simulink model "OpenLoopSpacecraft"  (Simulink 7.4)
settings: Solver=ode5  StartTime=0  StopTime=30  FixedStep=DeltaT  RelTol=1e-3
InitFcn:
  | %Bifocal Relay Mirror Spacecraft Dynamics Simulation          TA Sands
  | clear all;close all;clc;
  | 
  | %Constants0
  | Re=6371.2e3;mu=398601.2e9;          %earth radius and universal gravitation constant
  | 
  | %Spacecraft orbit
  | h=0;                                     %orbit altitude
  | R=Re+h;                             %orbit radius from center of earth
  | we=0.000072921158553;   %earth's angular velocity rad/solar sec(Vallado)
  | wo=sqrt(mu/(Re+h)^3);        %orbit angular velocity
  | incln=36.6001*pi/180;          %Inclination assumed Monterey Latitude
  | epsilon=12*pi/180;  alphao=0;
  | uo=0; nuo=0;                        %Start S/C beneath subsolar point
  | beta=60; gamma=1.5;
  | a=0.545491852; b=0.314939867;  c=0.704226952;   %Assumed spacecraft rectangular size
  | Area=[b*c a*c a*b];                 %projected area~m^2 in body x,y,z directions
  | density=4.39e-14;
  | kpre=-9.9639/24/3600/180*pi*0;      %nodal precession constant assumed zero here
  | wn=kpre*(Re/(Re+h))^3.5*cos(incln); %nodal precession (zero eccentricity)
  | V=wo*(Re+h);
  | rho=asin(Re/(h+Re));                %earth angular radius
  | Cd=2.5;     psun=4.5E-6;            %Drag coefficient and solar pressure constant~N/m^2
  | Kaero=-0.5*Cd*V^2;   Psolar=2*psun;  %constants for aero and solar torque calculation
  | dL=[0.002 0.002 0.008];             %predicted distance between cp and cg
  | Kme=2.3390e-005;
  | 
  | %Spacecraft Magnetic Properties (assumed)
  | mresid=[0 0 0.01];                  %Spacecraft residual magnetic moment
  | M=mresid;                           %Magnetic unit dipole vector
  | K=7.943e15;
  | 
  | %Spacecraft Inertia conditions
  | Ix=119.1259;   Iy=150.6615;   Iz=106.0288;  Ixy=-15.7678;  Iyz=22.31637;  Ixz=-6.54859;
  | Jact=[Ix Ixy Ixz;        Ixy  Iy  Iyz;       Ixz Iyz  Iz];                  %Moment of inertia matrix
  | 
  | Ix=90;   Iy=100;   Iz=250 ;   Ixy=10;  Iyz=-20;  Ixz=10;
  | Imo=[Ix Ixy Ixz;        Ixy  Iy  Iyz;       Ixz Iyz  Iz]                  %Moment of inertia matrix
  | %Jact=Imo
  | Iinv=(Imo)^-1                      %Moment of inertia inverse goes in dynamics block
  | 
  | %Spacecraft initial Euler state angles and rates
  | phio=0;thetao=0;psio=0;                    %Initial Euler Angles
  | phidoto=0;thetadoto=0;psidoto=0;     %Initial Euler Rates
  | 
  | %Calculation of initial quaternion (qo) and angular momentum (Ho)
  | s1=sin(phio/2);s2=sin(thetao/2);s3=sin(psio/2);c1=cos(phio/2);c2=cos(thetao/2);c3=cos(psio/2);
  | q1o=s1*c2*c3-c1*s2*s3;
  | q2o=c1*s2*c3+s1*c2*s3;              %Wie pg. 321
  | q3o=c1*c2*s3-s1*s2*c3;
  | q4o=c1*c2*c3+s1*s2*s3;
  | S1=sin(phio);S2=sin(thetao);S3=sin(psio);C1=cos(phio);C2=cos(thetao);C3=cos(psio);
  | wxo=phidoto-psidoto*S2-wo*S3*C2;
  | wyo=thetadoto*C1+psidoto*C2*S1-wo*(C3*C1+S3*S2*S1);
  | wzo=psidoto*C2*C1-thetadoto*S1-wo*(S3*S2*C1-C3*S1);
  | qo=[q1o q2o q3o q4o];
  | Ho=Imo*[wxo wyo wzo]';
  | norm(Ho)*1000;
  | 
  | %Calculate eclipse time for comparison with EPS calculations
  | Te=100.87*2*V/2/pi;
  | 
  | %CMG Properties (in degrees)
  | %beta=90*pi/180;                                     %Skew angle in degrees converted to radians
  | beta=[90;90;-90;0]; beta=beta.*pi./180;
  | 
  | Gimbal0=[-30*pi/180; 90*pi/180; -30*pi/180;0];   % Initial Gimbal angles for 0 H spin up
  | w_wheel=2800*(2*pi/60);                       %Wheel speed in RPM converted to rad/s
  | Iwheel=0.0614*1.3558179483314;        % Wheel inertia in slug-ft^2 converted (exact) to kg m^2
  | h_wheel=Iwheel*w_wheel;                     % CMG Wheel Angular Momentum
  | 
  | %PID Controller Gains
  | Kpx=100;   Kdx=300;   Kix=0;  Kpy=Kpx;   Kdy=Kdx;   Kiy=Kix;  Kpz=Kpx;   Kdz=Kdx;   Kiz=Kix;
  | %Kpx=10100;   Kdx=1.6*Kpx;   Kix=0;  Kpy=Kpx;   Kdy=Kdx;   Kiy=Kix;  Kpz=Kpx;   Kdz=Kdx;   Kiz=Kix;
  | Kff=-1;
  | roll=0;  pitch=0; yaw=30;   roll=roll*pi/180; pitch=pitch*pi/180; yaw=yaw*pi/180;
  | SlewTime=10;  Rate=40;   DeltaT=1/Rate;   SPUDengage=0 ; %yaw*180/pi/100000
  | 
  | % Adaptive feedforward parameters
  | ETA=7;  ETAc=1;
  | Ix=119.1259;   Iy=150.6615;   Iz=106.0288;  Ixy=-15.7678;  Iyz=22.31637;  Ixz=-6.54859; Imo;
  | Jhat0=[Ix Ixy Ixz;       Ixy  Iy  Iyz;       Ixz Iyz  Iz];
  | ThetaHat0=[Ix; Ixy; Ixz; Iy; Iyz; Iz; 0; 0; 0];
StopFcn:
  | figure(1);subplot(3,1,1);plot(t,JwdotCMD,'linewidth',2);grid;ylabel('FeedForward','fontname','time','fontsize',20)
  | title('FeedForward Trajectory No Disturbance','fontname','time','fontsize',20);legend('roll \phi','pitch \theta','yaw \psi')
  | subplot(3,1,2);plot(t,Jwdot,'linewidth',2);grid;ylabel('Output','fontname','time','fontsize',20)
  | subplot(3,1,3);plot(t,Jwdot-JwdotCMD,'linewidth',2);grid;ylabel('Trajectory Error','fontname','time','fontsize',20)
  | xlabel('time(sec)','fontname','time','fontsize',20);
libraries: aerospace x2, simulink x1
settings Model: Creator=tasands  LastModifiedBy=tasands
settings DataIOCC: SignalLoggingName=sigsOut
settings OptimizationCC: InlineInvariantSignals=on  InitFltsAndDblsToZero=on
settings DebuggingCC: SaveWithParameterizedLinksMsg=none  SignalResolutionControl=TryResolveAllWithWarning  SolverPrmCheckMsg=none  MultiTaskDSMMsg=warning  MultiTaskCondExecSysMsg=none  StrictBusMsg=None
settings HardwareCC: TargetHWDeviceType=32-bit Generic  ProdEqTarget=off
settings RTWCC: IncludeERTFirstTime=on
settings GRTTargetCC: TargetFcnLib=ansi_tfl_tmw.mat

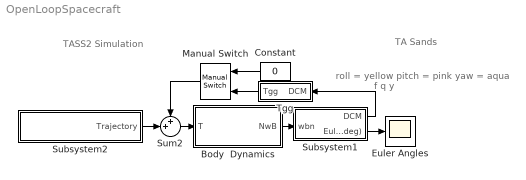
== system OpenLoopSpacecraft ==
  note: roll = yellow
      | pitch = pink
      | yaw = aqua
  note: TASS2 Simulation
  note: TA Sands
  note: f
      | q
      | y
  Body  Dynamics : Subsystem
      mask Display: disp('TASS2 Dynamics')
  Constant : Constant  Value=0  OutDataType=sfix(16)  OutScaling=2^0
  Euler Angles : Scope
      settings: TimeRange=30  YMin=-20  YMax=100
  Manual Switch : simulink/Signal Routing/Manual Switch  SystemSampleTime=-1  sw=1  action=0  varsize=off
  Subsystem1 : Subsystem
      mask Display: disp('Kinematics')
  Subsystem2 : Subsystem
      mask Display: disp('FeedForward Trajectory')
  Sum2 : Sum  Inputs=++|  OutDataType=sfix(16)  OutScaling=2^0  SaturateOnIntegerOverflow=on
  Tgg : Subsystem
      mask Display: disp('CG offet')
  wires:
  Body  Dynamics/1(NwB) -> Subsystem1/1(wbn)
  Subsystem1/1(DCM) -> Tgg/1(DCM)
  Subsystem1/2(Euler(deg)) -> Euler Angles/1
  Sum2/1 -> Body  Dynamics/1(T)
  Subsystem2/1(Trajectory) -> Sum2/2
  Manual Switch/1 -> Sum2/1
  Tgg/1(Tgg) -> Manual Switch/2
  Constant/1 -> Manual Switch/1

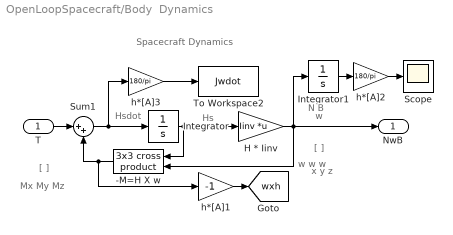
== system OpenLoopSpacecraft/Body  Dynamics ==
  note: w
  note: N B
  note: Hs
  note: Hsdot
  note: [ ]
  note: Mx
      | My
      | Mz
  note: [ ]
  note: w
      | w
      | w
  note: x
      | y
      | z
  note: Spacecraft Dynamics
  T : Inport  OutDataType=sfix(16)  OutScaling=2^0
  -M=H X w : aerospace/Axes Transformations/3x3 cross product  SystemSampleTime=-1
  H * Iinv : Gain  Gain=Iinv  Multiplication=Matrix(K*u)  ParameterDataType=sfix(16)  ParameterScaling=2^0  OutDataType=sfix(16)  OutScaling=2^0  SaturateOnIntegerOverflow=on  OutDataTypeStr=Inherit: Same as input  ParamDataTypeStr=Inherit: Same as input
  Integrator : Integrator
  Integrator1 : Integrator
  Scope : Scope
      settings: TimeRange=30  YMin=-50  YMax=200  SaveName=ScopeData5
  Sum1 : Sum  Inputs=|++  OutDataType=sfix(16)  OutScaling=2^0  SaturateOnIntegerOverflow=on  InputSameDT=on  OutDataTypeStr=Inherit: Same as first input
  To Workspace2 : ToWorkspace  VariableName=Jwdot  SampleTime=-1  SaveFormat=Array
  h*[A]1 : Gain  Gain=-1  ParameterDataType=sfix(16)  ParameterScaling=2^0  OutDataType=sfix(16)  OutScaling=2^0
  h*[A]2 : Gain  Gain=180/pi  ParameterDataType=sfix(16)  ParameterScaling=2^0  OutDataType=sfix(16)  OutScaling=2^0
  h*[A]3 : Gain  Gain=180/pi  ParameterDataType=sfix(16)  ParameterScaling=2^0  OutDataType=sfix(16)  OutScaling=2^0
  NwB : Outport  OutDataType=sfix(16)  OutScaling=2^0
  tag scope: wxh=global
  wires:
  Integrator/1 -> H * Iinv/1, -M=H X w/1
  H * Iinv/1 -> -M=H X w/2, Integrator1/1, NwB/1
  -M=H X w/1 -> Sum1/2, h*[A]1/1
  Sum1/1 -> Integrator/1, h*[A]3/1
  T/1 -> Sum1/1
  h*[A]1/1 -> [wxh]
  Integrator1/1 -> h*[A]2/1
  h*[A]2/1 -> Scope/1
  h*[A]3/1 -> To Workspace2/1

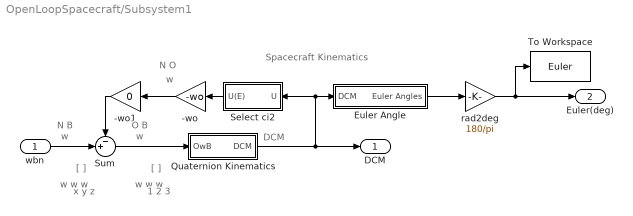
== system OpenLoopSpacecraft/Subsystem1 ==
  note: [ ]
  note: w
      | w
      | w
  note: x
      | y
      | z
  note: w
  note: N B
  note: w
  note: [ ]
  note: w
      | w
      | w
  note: 1
      | 2
      | 3
  note: w
  note: O B
  note: DCM
  note: N O
  note: Spacecraft Kinematics
  wbn : Inport  OutDataType=sfix(16)  OutScaling=2^0
  -wo : Gain  Gain=-wo  ParameterDataType=sfix(16)  ParameterScaling=2^0  OutDataType=sfix(16)  OutScaling=2^0  SaturateOnIntegerOverflow=on  OutDataTypeStr=Inherit: Same as input  ParamDataTypeStr=Inherit: Same as input
  -wo1 : Gain  Gain=0  ParameterDataType=sfix(16)  ParameterScaling=2^0  OutDataType=sfix(16)  OutScaling=2^0  SaturateOnIntegerOverflow=on  OutDataTypeStr=Inherit: Same as input  ParamDataTypeStr=Inherit: Same as input
  Euler Angle : Subsystem
  Quaternion Kinematics : Subsystem
  Select ci2 : Subsystem
  Sum : Sum  Inputs=-+|  OutDataType=sfix(16)  OutScaling=2^0  SaturateOnIntegerOverflow=on  InputSameDT=on  OutDataTypeStr=Inherit: Same as first input
  To Workspace : ToWorkspace  VariableName=Euler  SampleTime=-1  SaveFormat=Array
  rad2deg : Gain  Gain=180/pi  ParameterDataType=sfix(16)  ParameterScaling=2^0  OutDataType=sfix(16)  OutScaling=2^0  SaturateOnIntegerOverflow=on  OutDataTypeStr=Inherit: Same as input  ParamDataTypeStr=Inherit: Same as input
  DCM : Outport  OutDataType=sfix(16)  OutScaling=2^0
  Euler(deg) : Outport  Port=2  OutDataType=sfix(16)  OutScaling=2^0
  wires:
  Sum/1 -> Quaternion Kinematics/1(OwB)
  -wo/1 -> -wo1/1
  Select ci2/1(U(E)) -> -wo/1
  Quaternion Kinematics/1(DCM) -> Select ci2/1(U), Euler Angle/1(DCM), DCM/1
  -wo1/1 -> Sum/1
  wbn/1 -> Sum/2
  Euler Angle/1(Euler Angles) -> rad2deg/1
  rad2deg/1 -> Euler(deg)/1, To Workspace/1

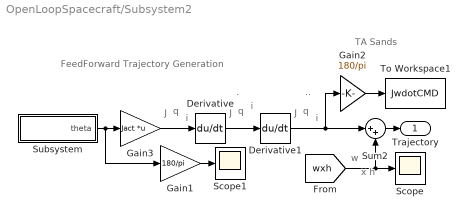
== system OpenLoopSpacecraft/Subsystem2 ==
  note: q
  note: ..
  note: q
  note: J
  note: w
  note: x h
  note: q
  note: .
  note: J
  note: TA Sands
  note: FeedForward Trajectory
      | Generation
  note: i
  note: i
  note: i
  note: J
  Derivative : Derivative
  Derivative1 : Derivative
  Gain1 : Gain  Gain=180/pi  ParameterDataType=sfix(16)  ParameterScaling=2^0  OutDataType=sfix(16)  OutScaling=2^0
  Gain2 : Gain  Gain=180/pi  ParameterDataType=sfix(16)  ParameterScaling=2^0  OutDataType=sfix(16)  OutScaling=2^0
  Gain3 : Gain  Gain=Jact  Multiplication=Matrix(K*u)  ParameterDataType=sfix(16)  ParameterScaling=2^0  OutDataType=sfix(16)  OutScaling=2^0
  Scope : Scope
      settings: TimeRange=30  YMin=-0.5  YMax=3  SaveName=ScopeData3
  Scope1 : Scope
      settings: TimeRange=30  YMin=0  YMax=30  SaveName=ScopeData4
  Subsystem : Subsystem
      mask Display: disp('Slew Angle')
  Sum2 : Sum  Inputs=|++  OutDataType=sfix(16)  OutScaling=2^0  SaturateOnIntegerOverflow=on
  To Workspace1 : ToWorkspace  VariableName=JwdotCMD  SampleTime=-1  SaveFormat=Array
  Trajectory : Outport  OutDataType=sfix(16)  OutScaling=2^0
  wires:
  Subsystem/1(theta) -> Gain1/1, Gain3/1
  Derivative/1 -> Derivative1/1
  Derivative1/1 -> Sum2/1, Gain2/1
  Sum2/1 -> Trajectory/1
  [wxh] -> Sum2/2, Scope/1
  Gain1/1 -> Scope1/1
  Gain3/1 -> Derivative/1
  Gain2/1 -> To Workspace1/1

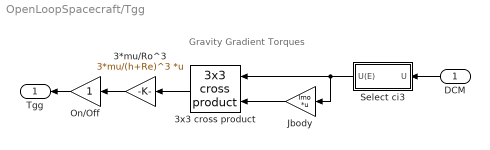
== system OpenLoopSpacecraft/Tgg ==
  note: Gravity Gradient Torques
  DCM : Inport  OutDataType=sfix(16)  OutScaling=2^0
  3*mu/Ro^3 : Gain  Gain=3*mu/(h+Re)^3  Multiplication=Matrix(K*u)  ParameterDataType=sfix(16)  ParameterScaling=2^0  OutDataType=sfix(16)  OutScaling=2^0  SaturateOnIntegerOverflow=on  OutDataTypeStr=Inherit: Same as input  ParamDataTypeStr=Inherit: Same as input
  3x3 cross product : aerospace/Axes Transformations/3x3 cross product  SystemSampleTime=-1
  Jbody : Gain  Gain=Imo  Multiplication=Matrix(K*u)  ParameterDataType=sfix(16)  ParameterScaling=2^0  OutDataType=sfix(16)  OutScaling=2^0  SaturateOnIntegerOverflow=on  OutDataTypeStr=Inherit: Same as input  ParamDataTypeStr=Inherit: Same as input
  On/Off : Gain  ParameterDataType=sfix(16)  ParameterScaling=2^0  OutDataType=sfix(16)  OutScaling=2^0  SaturateOnIntegerOverflow=on  OutDataTypeStr=Inherit: Same as input  ParamDataTypeStr=Inherit: Same as input
  Select ci3 : Subsystem
  Tgg : Outport  OutDataType=sfix(16)  OutScaling=2^0
  wires:
  Jbody/1 -> 3x3 cross product/2
  3*mu/Ro^3/1 -> On/Off/1
  3x3 cross product/1 -> 3*mu/Ro^3/1
  Select ci3/1(U(E)) -> 3x3 cross product/1, Jbody/1
  DCM/1 -> Select ci3/1(U)
  On/Off/1 -> Tgg/1

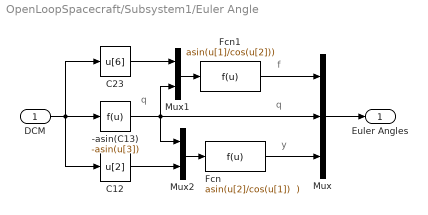
== system OpenLoopSpacecraft/Subsystem1/Euler Angle ==
  note: q
  note: f
  note: y
  note: q
  DCM : Inport  OutDataType=sfix(16)  OutScaling=2^0
  -asin(C13) : Fcn  Expr=-asin(u[3])
  C12 : Fcn  Expr=u[2]
  C23 : Fcn  Expr=u[6]
  Fcn : Fcn  Expr="asin(u[2]/cos(u[1])  )"
  Fcn1 : Fcn  Expr=asin(u[1]/cos(u[2]))
  Mux : Mux  Inputs=3
  Mux1 : Mux  Inputs=2
  Mux2 : Mux  Inputs=2
  Euler Angles : Outport  OutDataType=sfix(16)  OutScaling=2^0
  wires:
  C12/1 -> Mux2/2
  Fcn/1 -> Mux/3
  Mux2/1 -> Fcn/1
  C23/1 -> Mux1/1
  -asin(C13)/1 -> Mux2/1, Mux1/2, Mux/2
  Fcn1/1 -> Mux/1
  Mux1/1 -> Fcn1/1
  DCM/1 -> C12/1, C23/1, -asin(C13)/1
  Mux/1 -> Euler Angles/1

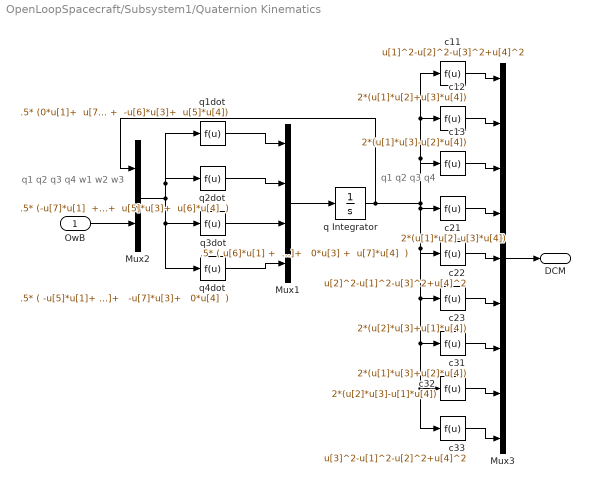
== system OpenLoopSpacecraft/Subsystem1/Quaternion Kinematics ==
  note: q1
      | q2
      | q3
      | q4
      | w1
      | w2
      | w3
  note: q1
      | q2
      | q3
      | q4
  OwB : Inport  OutDataType=sfix(16)  OutScaling=2^0
  Mux1 : Mux
  Mux2 : Mux  Inputs=2
  Mux3 : Mux  Inputs=9
  c11 : Fcn  Expr=u[1]^2-u[2]^2-u[3]^2+u[4]^2
  c12 : Fcn  Expr=2*(u[1]*u[2]+u[3]*u[4])
  c13 : Fcn  Expr=2*(u[1]*u[3]-u[2]*u[4])
  c21 : Fcn  Expr=2*(u[1]*u[2]-u[3]*u[4])
  c22 : Fcn  Expr=u[2]^2-u[1]^2-u[3]^2+u[4]^2
  c23 : Fcn  Expr=2*(u[2]*u[3]+u[1]*u[4])
  c31 : Fcn  Expr=2*(u[1]*u[3]+u[2]*u[4])
  c32 : Fcn  Expr=2*(u[2]*u[3]-u[1]*u[4])
  c33 : Fcn  Expr=u[3]^2-u[1]^2-u[2]^2+u[4]^2
  q Integrator : Integrator  InitialCondition=qo
  q1dot : Fcn  Expr=".5* (0*u[1]+  u[7]*u[2] +  -u[6]*u[3]+  u[5]*u[4])"
  q2dot : Fcn  Expr=".5* (-u[7]*u[1]  +  0*u[2]+  u[5]*u[3]+  u[6]*u[4]  )"
  q3dot : Fcn  Expr=".5* ( u[6]*u[1] +  -u[5]*u[2]+   0*u[3] +  u[7]*u[4]  )"
  q4dot : Fcn  Expr=".5* ( -u[5]*u[1]+   -u[6]*u[2]+   -u[7]*u[3]+   0*u[4]  )"
  DCM : Outport  OutDataType=sfix(16)  OutScaling=2^0
  wires:
  OwB/1 -> Mux2/2
  q1dot/1 -> Mux1/1
  q2dot/1 -> Mux1/2
  q3dot/1 -> Mux1/3
  q4dot/1 -> Mux1/4
  Mux1/1 -> q Integrator/1
  q Integrator/1 -> c13/1, c12/1, c11/1, c21/1, c22/1, c23/1, c31/1, c33/1, c32/1, Mux2/1
  c11/1 -> Mux3/1
  c12/1 -> Mux3/2
  c13/1 -> Mux3/3
  c22/1 -> Mux3/5
  c21/1 -> Mux3/4
  c23/1 -> Mux3/6
  c31/1 -> Mux3/7
  c32/1 -> Mux3/8
  c33/1 -> Mux3/9
  Mux3/1 -> DCM/1
  Mux2/1 -> q2dot/1, q1dot/1, q3dot/1, q4dot/1

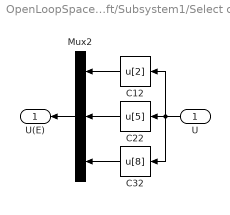
== system OpenLoopSpacecraft/Subsystem1/Select ci2 ==
  U : Inport  OutDataType=sfix(16)  OutScaling=2^0
  C12 : Fcn  Expr=u[2]
  C22 : Fcn  Expr=u[5]
  C32 : Fcn  Expr=u[8]
  Mux2 : Mux  Inputs=3
  U(E) : Outport  OutDataType=sfix(16)  OutScaling=2^0
  wires:
  C12/1 -> Mux2/1
  C22/1 -> Mux2/2
  C32/1 -> Mux2/3
  U/1 -> C32/1, C22/1, C12/1
  Mux2/1 -> U(E)/1

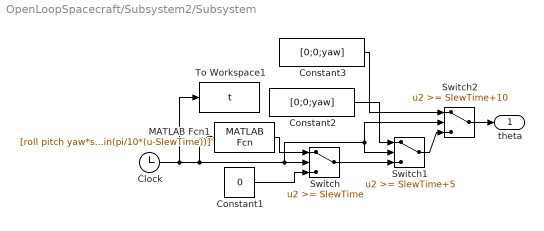
== system OpenLoopSpacecraft/Subsystem2/Subsystem ==
  Clock : Clock
      settings: Decimation=10
  Constant1 : Constant  Value=0  OutDataType=sfix(16)  OutScaling=2^0
  Constant2 : Constant  Value=[0;0;yaw]  OutDataType=sfix(16)  OutScaling=2^0
  Constant3 : Constant  Value=[0;0;yaw]  OutDataType=sfix(16)  OutScaling=2^0
  MATLAB Fcn1 : MATLABFcn  MATLABFcn=[roll pitch yaw*sin(pi/10*(u-SlewTime))]'
  Switch : Switch  Threshold=SlewTime
  Switch1 : Switch  Threshold=SlewTime+5
  Switch2 : Switch  Threshold=SlewTime+10
  To Workspace1 : ToWorkspace  VariableName=t  SampleTime=-1  SaveFormat=Array
  theta : Outport  OutDataType=sfix(16)  OutScaling=2^0
  wires:
  Switch/1 -> Switch1/3
  Constant1/1 -> Switch/3
  Clock/1 -> Switch/2, Switch1/2, Switch2/2, MATLAB Fcn1/1, To Workspace1/1
  MATLAB Fcn1/1 -> Switch/1
  Constant2/1 -> Switch1/1
  Switch1/1 -> Switch2/3
  Switch2/1 -> theta/1
  Constant3/1 -> Switch2/1

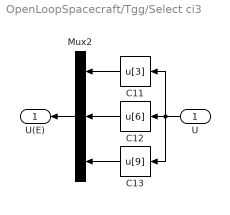
== system OpenLoopSpacecraft/Tgg/Select ci3 ==
  U : Inport  OutDataType=sfix(16)  OutScaling=2^0
  C11 : Fcn  Expr=u[3]
  C12 : Fcn  Expr=u[6]
  C13 : Fcn  Expr=u[9]
  Mux2 : Mux  Inputs=3
  U(E) : Outport  OutDataType=sfix(16)  OutScaling=2^0
  wires:
  Mux2/1 -> U(E)/1
  U/1 -> C13/1, C11/1, C12/1
  C13/1 -> Mux2/3
  C12/1 -> Mux2/2
  C11/1 -> Mux2/1
